simulink model "Vienna_sogi_curcon1"  (R2022b)
settings: Solver=ode23t  StartTime=0.0  StopTime=0.1  RelTol=1e-3
undefined symbols (not defined in the file): acdc, Cur_loop_upper_limit_acdc, DiscIntNeverNeededParam, Tsim, vdc_fbk_filter
libraries: simulink x9, spsDiodeLib x6, spsMosfetLib x6, spsSeriesRLCBranchLib x5, spsVoltageMeasurementLib x4, spsMeanLib x4, spsCurrentMeasurementLib x3, spsControlledVoltageSourceLib x3, spsRMSLib x2, spsThreePhaseSourceLib x1, spsTHDLib x1, spsTriangleGeneratorLib x1
(part 2 of 2)

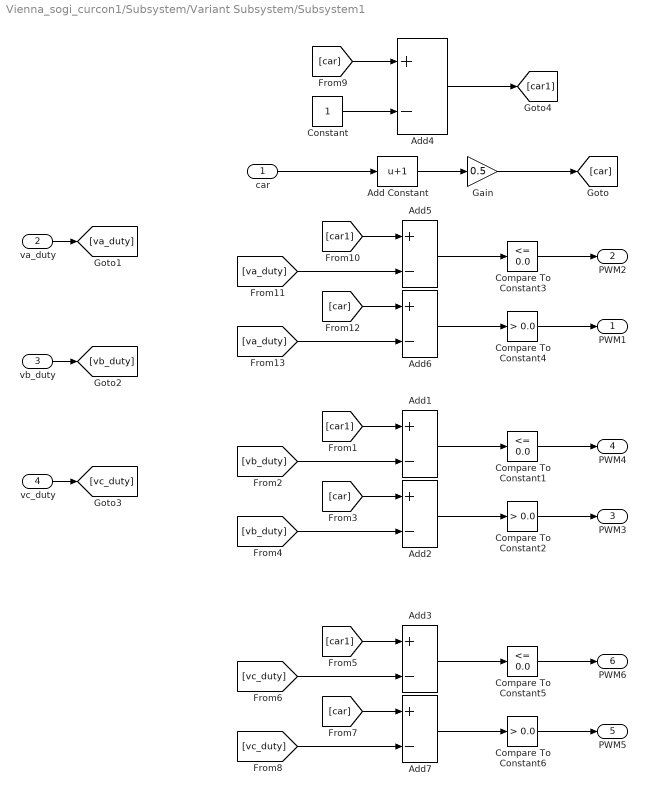
== system Vienna_sogi_curcon1/Subsystem/Variant Subsystem/Subsystem1 ==
  car : Inport
  va_duty : Inport  Port=2
  vb_duty : Inport  Port=3
  vc_duty : Inport  Port=4
  Add Constant : Bias  Bias=1  SaturateOnIntegerOverflow=off
  Add{1..7} (7 alike) : Sum  Inputs=+-
  Compare To Constant1 : simulink/Logic and Bit Operations/Compare To Constant  relop=<=  const=0.0  OutDataTypeStr=boolean
  Compare To Constant2 : simulink/Logic and Bit Operations/Compare To Constant  relop=>  const=0.0  OutDataTypeStr=boolean
  Compare To Constant3 : simulink/Logic and Bit Operations/Compare To Constant  relop=<=  const=0.0  OutDataTypeStr=boolean
  Compare To Constant4 : simulink/Logic and Bit Operations/Compare To Constant  relop=>  const=0.0  OutDataTypeStr=boolean
  Compare To Constant5 : simulink/Logic and Bit Operations/Compare To Constant  relop=<=  const=0.0  OutDataTypeStr=boolean
  Compare To Constant6 : simulink/Logic and Bit Operations/Compare To Constant  relop=>  const=0.0  OutDataTypeStr=boolean
  Constant : Constant
  Gain : Gain  Gain=0.5
  PWM1 : Outport
  PWM2 : Outport  Port=2
  PWM3 : Outport  Port=3
  PWM4 : Outport  Port=4
  PWM5 : Outport  Port=5
  PWM6 : Outport  Port=6
  wires:
  Add6/1 -> Compare To Constant4/1
  [va_duty] -> Add5/2
  va_duty/1 -> [va_duty]
  vb_duty/1 -> [vb_duty]
  [car1] -> Add5/1
  Compare To Constant3/1 -> PWM2/1
  Add Constant/1 -> Gain/1
  car/1 -> Add Constant/1
  vc_duty/1 -> [vc_duty]
  Add5/1 -> Compare To Constant3/1
  Add4/1 -> [car1]
  [va_duty] -> Add6/2
  Compare To Constant4/1 -> PWM1/1
  [car] -> Add4/1
  Gain/1 -> [car]
  Constant/1 -> Add4/2
  [car] -> Add6/1
  Add2/1 -> Compare To Constant2/1
  [vb_duty] -> Add1/2
  Add1/1 -> Compare To Constant1/1
  [car] -> Add2/1
  [vb_duty] -> Add2/2
  [car1] -> Add1/1
  Add7/1 -> Compare To Constant6/1
  [vc_duty] -> Add3/2
  Add3/1 -> Compare To Constant5/1
  [car] -> Add7/1
  [vc_duty] -> Add7/2
  [car1] -> Add3/1
  Compare To Constant1/1 -> PWM4/1
  Compare To Constant2/1 -> PWM3/1
  Compare To Constant5/1 -> PWM6/1
  Compare To Constant6/1 -> PWM5/1

== system Vienna_sogi_curcon1/CurrentController1/Variant Subsystem/PR/PRcontroller ==
  In1 : Inport
  Add : Sum
  Discrete Transfer Fcn : DiscreteTransferFcn  Numerator=acdc.PR_num  Denominator=acdc.PR_den
  Gain : Gain  Gain=acdc.cur_con_kp
  Gain1 : Gain  Gain=acdc.cur_con_ki
  Saturation : Saturate  UpperLimit=Cur_loop_upper_limit_acdc  LowerLimit=-Cur_loop_upper_limit_acdc
  ia_duty1 : Outport
  wires:
  Saturation/1 -> ia_duty1/1
  In1/1 -> Gain1/1, Gain/1
  Add/1 -> Saturation/1
  Gain1/1 -> Discrete Transfer Fcn/1
  Discrete Transfer Fcn/1 -> Add/2
  Gain/1 -> Add/1

== system Vienna_sogi_curcon1/CurrentController1/Variant Subsystem/PR/PRcontroller1 ==
  In1 : Inport
  Add : Sum
  Discrete Transfer Fcn : DiscreteTransferFcn  Numerator=acdc.PR_num  Denominator=acdc.PR_den
  Gain : Gain  Gain=acdc.cur_con_kp
  Gain1 : Gain  Gain=acdc.cur_con_ki
  Saturation : Saturate  UpperLimit=Cur_loop_upper_limit_acdc  LowerLimit=-Cur_loop_upper_limit_acdc
  va_pol1 : Outport
  wires:
  Saturation/1 -> va_pol1/1
  In1/1 -> Gain1/1, Gain/1
  Add/1 -> Saturation/1
  Gain1/1 -> Discrete Transfer Fcn/1
  Discrete Transfer Fcn/1 -> Add/2
  Gain/1 -> Add/1

== system Vienna_sogi_curcon1/CurrentController1/Variant Subsystem/PR/PRcontroller2 ==
  In1 : Inport
  Add : Sum
  Discrete Transfer Fcn : DiscreteTransferFcn  Numerator=acdc.PR_num  Denominator=acdc.PR_den
  Gain : Gain  Gain=acdc.cur_con_kp
  Gain1 : Gain  Gain=acdc.cur_con_ki
  Saturation : Saturate  UpperLimit=Cur_loop_upper_limit_acdc  LowerLimit=-Cur_loop_upper_limit_acdc
  vb_pol1 : Outport
  wires:
  Saturation/1 -> vb_pol1/1
  In1/1 -> Gain1/1, Gain/1
  Add/1 -> Saturation/1
  Gain1/1 -> Discrete Transfer Fcn/1
  Discrete Transfer Fcn/1 -> Add/2
  Gain/1 -> Add/1

== system Vienna_sogi_curcon1/CurrentController1/Variant Subsystem/SOGI_PR/PRcontroller1 ==
  In1 : Inport
  w_est : Inport  Port=2
  Add : Sum
  Gain : Gain  Gain=acdc.cur_con_kp
  Gain1 : Gain  Gain=acdc.cur_con_ki
  Saturation : Saturate  UpperLimit=Cur_loop_upper_limit_acdc  LowerLimit=-Cur_loop_upper_limit_acdc
  Subsystem : Subsystem
  ia_duty1 : Outport
  wires:
  Saturation/1 -> ia_duty1/1
  In1/1 -> Gain/1, Gain1/1
  Add/1 -> Saturation/1
  Gain1/1 -> Subsystem/1(Val)
  Subsystem/1(v) -> Add/2
  Gain/1 -> Add/1
  w_est/1 -> Subsystem/2(w_est)

== system Vienna_sogi_curcon1/CurrentController1/Variant Subsystem/SOGI_PR/PRcontroller2 ==
  In1 : Inport
  w_est : Inport  Port=2
  Add : Sum
  Gain : Gain  Gain=acdc.cur_con_kp
  Gain1 : Gain  Gain=acdc.cur_con_ki
  Saturation : Saturate  UpperLimit=Cur_loop_upper_limit_acdc  LowerLimit=-Cur_loop_upper_limit_acdc
  Subsystem : Subsystem
  ia_duty1 : Outport
  wires:
  Saturation/1 -> ia_duty1/1
  In1/1 -> Gain/1, Gain1/1
  Add/1 -> Saturation/1
  Gain1/1 -> Subsystem/1(Val)
  Subsystem/1(v) -> Add/2
  Gain/1 -> Add/1
  w_est/1 -> Subsystem/2(w_est)

== system Vienna_sogi_curcon1/CurrentController1/Variant Subsystem/SOGI_PR/PRcontroller3 ==
  In1 : Inport
  w_est : Inport  Port=2
  Add : Sum
  Gain : Gain  Gain=acdc.cur_con_kp
  Gain1 : Gain  Gain=acdc.cur_con_ki
  Saturation : Saturate  UpperLimit=Cur_loop_upper_limit_acdc  LowerLimit=-Cur_loop_upper_limit_acdc
  Subsystem : Subsystem
  ia_duty1 : Outport
  wires:
  Saturation/1 -> ia_duty1/1
  In1/1 -> Gain/1, Gain1/1
  Add/1 -> Saturation/1
  Gain1/1 -> Subsystem/1(Val)
  Subsystem/1(v) -> Add/2
  Gain/1 -> Add/1
  w_est/1 -> Subsystem/2(w_est)

== system Vienna_sogi_curcon1/PLL1/Subsystem/SOGI/Subsystem ==
  Val : Inport
  w_est : Inport  Port=2
  Add : Sum  Inputs=+-
  Add1 : Sum  Inputs=-+
  Delay2 : Delay  DelayLength=1
  Discrete-Time Integrator : DiscreteIntegrator  SampleTime=-1  ICPrevOutput=DiscIntNeverNeededParam  ICPrevScaledInput=DiscIntNeverNeededParam
  Discrete-Time Integrator1 : DiscreteIntegrator  SampleTime=-1  ICPrevOutput=DiscIntNeverNeededParam  ICPrevScaledInput=DiscIntNeverNeededParam
  Gain : Gain  Gain=acdc.sogi_k
  Product : Product
  Product1 : Product
  v : Outport
  qv : Outport  Port=2
  wires:
  Discrete-Time Integrator1/1 -> Product1/2
  w_est/1 -> Product1/1, Product/2
  Gain/1 -> Add/1
  Val/1 -> Add1/2
  Discrete-Time Integrator/1 -> v/1, Discrete-Time Integrator1/1, Add1/1
  Add1/1 -> Gain/1
  Add/1 -> Product/1
  Product1/1 -> qv/1, Delay2/1
  Product/1 -> Discrete-Time Integrator/1
  Delay2/1 -> Add/2

== system Vienna_sogi_curcon1/PLL1/Subsystem/SOGI/Subsystem1 ==
  Val : Inport
  w_est : Inport  Port=2
  Add : Sum  Inputs=+-
  Add1 : Sum  Inputs=-+
  Delay2 : Delay  DelayLength=1
  Discrete-Time Integrator : DiscreteIntegrator  SampleTime=-1  ICPrevOutput=DiscIntNeverNeededParam  ICPrevScaledInput=DiscIntNeverNeededParam
  Discrete-Time Integrator1 : DiscreteIntegrator  SampleTime=-1  ICPrevOutput=DiscIntNeverNeededParam  ICPrevScaledInput=DiscIntNeverNeededParam
  Gain : Gain  Gain=acdc.sogi_k
  Product : Product
  Product1 : Product
  v : Outport
  qv : Outport  Port=2
  wires:
  Discrete-Time Integrator1/1 -> Product1/2
  w_est/1 -> Product1/1, Product/2
  Gain/1 -> Add/1
  Val/1 -> Add1/2
  Discrete-Time Integrator/1 -> v/1, Discrete-Time Integrator1/1, Add1/1
  Add1/1 -> Gain/1
  Add/1 -> Product/1
  Product1/1 -> qv/1, Delay2/1
  Product/1 -> Discrete-Time Integrator/1
  Delay2/1 -> Add/2

== system Vienna_sogi_curcon1/CurrentController1/Variant Subsystem/SOGI_PR/PRcontroller1/Subsystem ==
  Val : Inport
  w_est : Inport  Port=2
  Add : Sum  Inputs=+-
  Add1 : Sum  Inputs=-+
  Delay2 : Delay  DelayLength=1
  Discrete-Time Integrator : DiscreteIntegrator  SampleTime=-1  ICPrevOutput=DiscIntNeverNeededParam  ICPrevScaledInput=DiscIntNeverNeededParam
  Discrete-Time Integrator1 : DiscreteIntegrator  SampleTime=-1  ICPrevOutput=DiscIntNeverNeededParam  ICPrevScaledInput=DiscIntNeverNeededParam
  Gain : Gain  Gain=acdc.cur_con_sogi_k
  Product : Product
  Product1 : Product
  v : Outport
  qv : Outport  Port=2
  wires:
  Discrete-Time Integrator1/1 -> Product1/2
  w_est/1 -> Product1/1, Product/2
  Gain/1 -> Add/1
  Val/1 -> Add1/2
  Discrete-Time Integrator/1 -> v/1, Discrete-Time Integrator1/1, Add1/1
  Add1/1 -> Gain/1
  Add/1 -> Product/1
  Product1/1 -> qv/1, Delay2/1
  Product/1 -> Discrete-Time Integrator/1
  Delay2/1 -> Add/2

== system Vienna_sogi_curcon1/CurrentController1/Variant Subsystem/SOGI_PR/PRcontroller2/Subsystem ==
  Val : Inport
  w_est : Inport  Port=2
  Add : Sum  Inputs=+-
  Add1 : Sum  Inputs=-+
  Delay2 : Delay  DelayLength=1
  Discrete-Time Integrator : DiscreteIntegrator  SampleTime=-1  ICPrevOutput=DiscIntNeverNeededParam  ICPrevScaledInput=DiscIntNeverNeededParam
  Discrete-Time Integrator1 : DiscreteIntegrator  SampleTime=-1  ICPrevOutput=DiscIntNeverNeededParam  ICPrevScaledInput=DiscIntNeverNeededParam
  Gain : Gain  Gain=acdc.cur_con_sogi_k
  Product : Product
  Product1 : Product
  v : Outport
  qv : Outport  Port=2
  wires:
  Discrete-Time Integrator1/1 -> Product1/2
  w_est/1 -> Product1/1, Product/2
  Gain/1 -> Add/1
  Val/1 -> Add1/2
  Discrete-Time Integrator/1 -> v/1, Discrete-Time Integrator1/1, Add1/1
  Add1/1 -> Gain/1
  Add/1 -> Product/1
  Product1/1 -> qv/1, Delay2/1
  Product/1 -> Discrete-Time Integrator/1
  Delay2/1 -> Add/2

== system Vienna_sogi_curcon1/CurrentController1/Variant Subsystem/SOGI_PR/PRcontroller3/Subsystem ==
  Val : Inport
  w_est : Inport  Port=2
  Add : Sum  Inputs=+-
  Add1 : Sum  Inputs=-+
  Delay2 : Delay  DelayLength=1
  Discrete-Time Integrator : DiscreteIntegrator  SampleTime=-1  ICPrevOutput=DiscIntNeverNeededParam  ICPrevScaledInput=DiscIntNeverNeededParam
  Discrete-Time Integrator1 : DiscreteIntegrator  SampleTime=-1  ICPrevOutput=DiscIntNeverNeededParam  ICPrevScaledInput=DiscIntNeverNeededParam
  Gain : Gain  Gain=acdc.cur_con_sogi_k
  Product : Product
  Product1 : Product
  v : Outport
  qv : Outport  Port=2
  wires:
  Discrete-Time Integrator1/1 -> Product1/2
  w_est/1 -> Product1/1, Product/2
  Gain/1 -> Add/1
  Val/1 -> Add1/2
  Discrete-Time Integrator/1 -> v/1, Discrete-Time Integrator1/1, Add1/1
  Add1/1 -> Gain/1
  Add/1 -> Product/1
  Product1/1 -> qv/1, Delay2/1
  Product/1 -> Discrete-Time Integrator/1
  Delay2/1 -> Add/2

== matlab function Vienna_sogi_curcon1/PLL1/Subsystem4/MATLAB Function3 ==
  data: th_a input; sin_a output size=1; sin_b output; sin_c output
function [sin_a,sin_b,sin_c]  = fcn(th_a)

sin_a =  sin(th_a);
sin_b =  sin(th_a - 2*pi/3);
sin_c =  sin(th_a + 2*pi/3);

== matlab function Vienna_sogi_curcon1/PLL1/Subsystem4/MATLAB Function7 ==
  data: al input; be input; d output; th input; q output; o output
function [d,q,o] = fcn(al,be,th)


% d = cos(th)*al + sin(th)*be;
% q = -sin(th)*al +cos(th)*be;
% o =0;


q = cos(th)*al + sin(th)*be;
d = -(-sin(th)*al +cos(th)*be);
o =0;

== matlab function Vienna_sogi_curcon1/Subsystem2/MATLAB Function1 ==
  data: Pin input; Pout input; Eff output; VA input; PF output
function [Eff,PF]  = fcn(Pin,Pout,VA)

if(Pin > 0.0001)
        Eff = Pout/Pin;
else

     Eff = 0;
end

if(Pin > 0.0001)
        PF = Pin/VA;
else

     PF = 0;
end

== matlab function Vienna_sogi_curcon1/Vbus_Controller/MATLAB Function4 ==
  data: vdc_max input; Tcon input; vdc_ref output; vdc_old input
function vdc_ref  = fcn(vdc_max,Tcon,vdc_old)


vdc_ref =  vdc_old + 8000*Tcon;



if(vdc_ref > vdc_max)
    ved_ref = vdc_max;
end

== matlab function Vienna_sogi_curcon1/PLL1/Subsystem4/MATLAB Function2 ==
  data: we input; Ts input; th_out output size=1; th_in input
function th_out  = fcn(we,Ts,th_in)


    th = th_in + we*Ts; 

    if(th > 2*pi)
        th_out = th -2*pi;
    elseif(th < 0.0)
        th_out = abs(th);
    else
        th_out = th;
    end

== matlab function Vienna_sogi_curcon1/Current Ref Generation/Variant Subsystem/power control/MATLAB Function4 ==
  data: va input; vb input; ia output; ib output; ic output; vc input; Pin input
function [ia,ib,ic] = fcn(va,vb,vc,Pin)


v_al = sqrt(2/3)*(va - vb/2 - vc/2);
v_be = sqrt(2/3)*(0 + sqrt(3)*vb/2 - sqrt(3)*vc/2);
v_ga = sqrt(2/3)*(va/2 + vb/2  + vc/2);

i_al = v_al*Pin/ (v_al^2 + v_be^2);
i_be = v_be*Pin/ (v_al^2 + v_be^2);


ia =  sqrt(2/3)*i_al;
ib =  sqrt(2/3)*( -i_al/2 + sqrt(3)/2*i_be);
ic =  sqrt(2/3)*( -i_al/2 - sqrt(3)/2*i_be);

== matlab function Vienna_sogi_curcon1/Current Ref Generation/Variant Subsystem/power control seq comp/MATLAB Function1 ==
  data: al input; be input; a output; b output; c output
function [a,b,c] = fcn(al,be)


a = al;
b = -1/2*al + sqrt(3)/2*be;
c = -1/2*al - sqrt(3)/2*be;

== matlab function Vienna_sogi_curcon1/PLL1/Subsystem/SOGI/MATLAB Function4 ==
  data: a input; b input; c input; al output; be output; ga output
function [al,be,ga] = fcn(a,b,c)


al = 2/3*(a - b/2 - c/2);
be = 2/3*(0 + sqrt(3)*b/2 - sqrt(3)*c/2);
ga = 2/3*(a/2 + b/2  + c/2);

== matlab function Vienna_sogi_curcon1/Current Ref Generation/Variant Subsystem/power control seq comp/MATLAB Function3 ==
  data: v_al_p input; i_al output size=1; i_be output; v_be_p input; v_al_n input; v_be_n input; p_ref input
function [i_al,i_be]  = fcn(v_al_p,v_be_p,v_al_n,v_be_n,p_ref)


fact = (p_ref*2/3)/(v_al_p^2 + v_be_p^2 - v_al_n^2 - v_be_n^2);

i_al_p  = v_al_p*fact;
i_be_p  = v_be_p*fact;
i_al_n  = -v_al_n*fact;
i_be_n  = -v_be_n*fact;

i_al = i_al_p + i_al_n;
i_be = i_be_p + i_be_n;
